simulink model "Part1_new"  (R2023b)
settings: Solver=ode23t  StartTime=0.0  StopTime=2  MaxStep=0.2  RelTol=1e-3
model workspace (MATLAB code in the model file):
  | m = 0.1;
  | d = 0.5;
  | k = 8;
libraries: fl_lib x29, nesl_utility x18
settings Model: Creator=oscar  LastModifiedBy=elliot
settings RTWCC: GPUComputeCapability=5.0

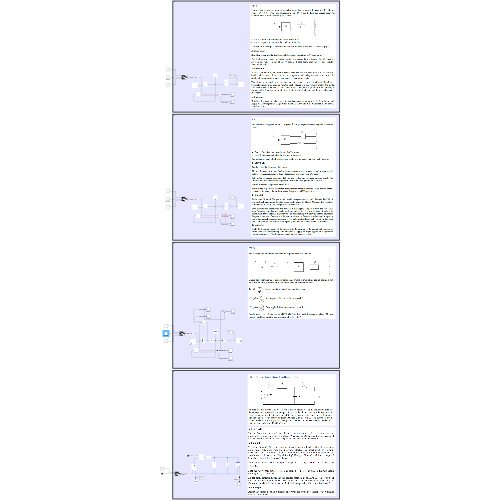
[thumbnail: Simulink's stored preview of the top-level diagram]
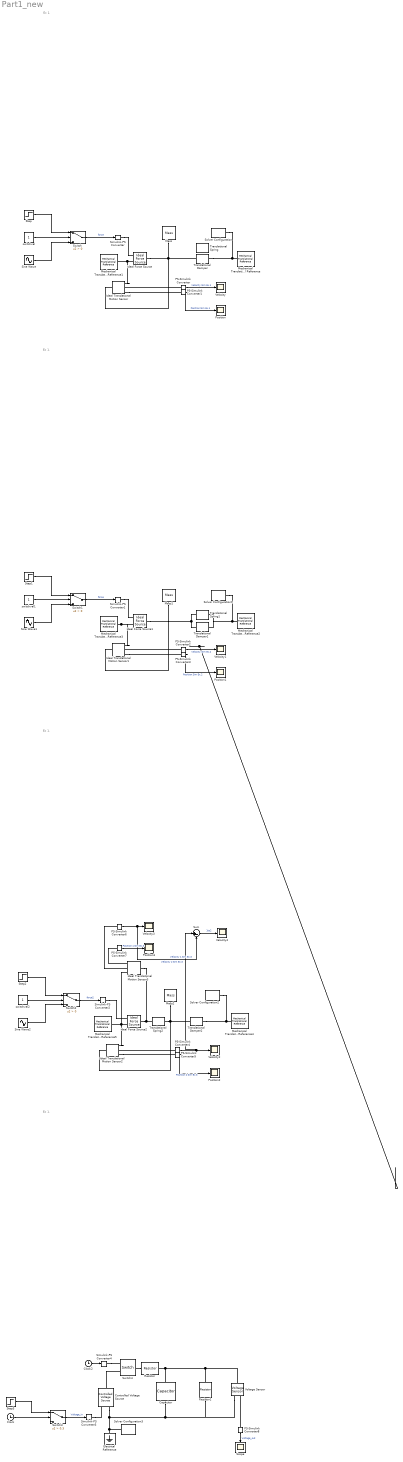
== system Part1_new ==
  note: Ex 1.
  note: Ex 1.
  note: Ex 1.
  note: Ex 1.
  Capacitor : fl_lib/Electrical/Electrical Elements/Capacitor  c=10 F  r=1e-6 Ohm  g=0 1/Ohm  i_specify=off  i_priority=None  i=0 A  i_nominal_specify=off  i_nominal_unit=A  i_nominal_value=1  v_specify=off  v_priority=None  v=0 V  v_nominal_specify=off  v_nominal_unit=V  v_nominal_value=1  vc_specify=off  vc_priority=High  vc=0 V  vc_nominal_specify=off  vc_nominal_unit=V  vc_nominal_value=1
  Clock : Clock
  Clock2 : Clock
  Controlled Voltage Source : fl_lib/Electrical/Electrical Sources/Controlled Voltage Source
  Electrical Reference : fl_lib/Electrical/Electrical Elements/Electrical Reference
  Ideal Force Source : fl_lib/Mechanical/Mechanical Sources/Ideal Force Source
  Ideal Force Source1 : fl_lib/Mechanical/Mechanical Sources/Ideal Force Source
  Ideal Force Source2 : fl_lib/Mechanical/Mechanical Sources/Ideal Force Source
  Ideal Translational Motion Sensor{,1..3} (4 alike) : fl_lib/Mechanical/Mechanical Sensors/Ideal Translational Motion Sensor  reference=foundation.enum.MeasurementReference.difference  acceleration_port=false  velocity_port=true  position_port=true  offset=0 m
  Mass : fl_lib/Mechanical/Translational Elements/Mass  mass=m kg  num_ports=foundation.enum.numPorts2.one  v_specify=off  v_priority=High  v=0 m/s  v_nominal_specify=off  v_nominal_unit=m/s  v_nominal_value=1  f_specify=off  f_priority=None  f=0 N  f_nominal_specify=off  f_nominal_unit=N  f_nominal_value=1
  Mass1 : fl_lib/Mechanical/Translational Elements/Mass  mass=m kg  num_ports=foundation.enum.numPorts2.one  v_specify=off  v_priority=High  v=0 m/s  v_nominal_specify=off  v_nominal_unit=m/s  v_nominal_value=1  f_specify=off  f_priority=None  f=0 N  f_nominal_specify=off  f_nominal_unit=N  f_nominal_value=1
  Mass2 : fl_lib/Mechanical/Translational Elements/Mass  mass=m kg  num_ports=foundation.enum.numPorts2.one  v_specify=off  v_priority=High  v=0 m/s  v_nominal_specify=off  v_nominal_unit=m/s  v_nominal_value=1  f_specify=off  f_priority=None  f=0 N  f_nominal_specify=off  f_nominal_unit=N  f_nominal_value=1
  Mechanical Translational Reference{,1..5} (6 alike) : fl_lib/Mechanical/Translational Elements/Mechanical Translational Reference
  PS-Simulink Converter{,1..8} (9 alike) : nesl_utility/PS-Simulink Converter  PhysicalDomain=network_engine_domain  SubClassName=ps_output  LeftPortType=input  RightPortType=output  PseudoPeriodic=off  Frequencies=[]  VectorFormat=inherit  Unit=inherit  AffineConversion=off
  Position{,1..3} (4 alike) : Scope
  Resistor : fl_lib/Electrical/Electrical Elements/Resistor  R=200 Ohm  i_specify=off  i_priority=None  i=0 A  i_nominal_specify=off  i_nominal_unit=A  i_nominal_value=1  v_specify=off  v_priority=None  v=0 V  v_nominal_specify=off  v_nominal_unit=V  v_nominal_value=1
  Resistor1 : fl_lib/Electrical/Electrical Elements/Resistor  R=200 Ohm  i_specify=off  i_priority=None  i=0 A  i_nominal_specify=off  i_nominal_unit=A  i_nominal_value=1  v_specify=off  v_priority=None  v=0 V  v_nominal_specify=off  v_nominal_unit=V  v_nominal_value=1
  Scope : Scope
  Simulink-PS Converter{,1,3..4} (4 alike) : nesl_utility/Simulink-PS Converter  PhysicalDomain=network_engine_domain  SubClassName=ps_input  LeftPortType=input  RightPortType=output  PseudoPeriodic=off  Frequencies=[]  NoiseDistribution=none  NoiseParameters=[]  Unit=1  AffineConversion=off  FilteringAndDerivatives=provide  SimscapeFilterOrder=1  InputFilterTimeConstant=0.001  UdotUserProvided=0
  Simulink-PS Converter2 : nesl_utility/Simulink-PS Converter  PhysicalDomain=network_engine_domain  SubClassName=ps_input  LeftPortType=input  RightPortType=output  PseudoPeriodic=off  Frequencies=[]  NoiseDistribution=none  NoiseParameters=[]  Unit=1  AffineConversion=off  FilteringAndDerivatives=filter  SimscapeFilterOrder=1  InputFilterTimeConstant=0.001  UdotUserProvided=0
  Sine Wave : Sin  Frequency=10  SampleTime=0
  Sine Wave1 : Sin  Frequency=10  SampleTime=0
  Sine Wave2 : Sin  Frequency=10  SampleTime=0
  Solver Configuration{,1..3} (4 alike) : nesl_utility/Solver Configuration  PhysicalDomain=network_engine_domain  SubClassName=solver  LeftPortType=input  RightPortType=generic  Tones=[]  Harmonics=[]  SimulateNoise=off  Profile=off  UseLocalSampling=off  EnableSwitchedLinearOptims=on  FrequencyDomain=off  UseCCode=off  RelTol=0.001  AbsTol=0.001  MinStep=1e-09  ToWorkspace=off  RevertToSquareIcSolve=off  NumHomotopyIterations=100  PhasorMode=off  PhasorModeNumHarmonics=1  ConsistencySolver=NEWTON_XTOL_AFTER_FTOL  IndexReductionMethod=DerivativeReplacement  DoDC=off  ResidualTolerance=1e-09  ConsistencyTolSource=GLOBAL  ConsistencyAbsTol=0.001  ConsistencyRelTol=0.001  ConsistencyTolFactor=0.001  UseLocalSolver=off  LocalSolverChoice=NE_BACKWARD_EULER_ADVANCER  ResolveIndetEquations=on  FunctionEvalNumThread=1  LocalSolverSampleTime=0.001  DoFixedCost=off  MaxNonlinIter=3  MaxModeIter=2  ComputeImpulses=off  ImpulseIterations=2  LinearAlgebra=auto  LinearAlgebraNumThread=0  EquationFormulation=NE_TIME_EF  DelaysMemoryBudget=1024  AutomaticFiltering=on  FilteringTimeConstant=0.001  PartitionStorageMethod=AS_NEEDED  PartitionMemoryBudget=1024  PartitionMethod=ROBUST  MultibodyUseLocalSolver=off  MultibodyLocalSolverChoice=ODE1  MultibodyLocalSolverSampleTime=0.001
  Step : Step  Time=0  SampleTime=0
  Step1 : Step  Time=0  SampleTime=0
  Step2 : Step  Time=0  SampleTime=0
  Step3 : Step  Time=0  After=12  SampleTime=0
  Sum : Sum  Inputs=|+-
  Switch : Switch  Criteria=u2 > Threshold  SaturateOnIntegerOverflow=off  InputSameDT=off
  Switch1 : Switch  Criteria=u2 > Threshold  SaturateOnIntegerOverflow=off  InputSameDT=off
  Switch2 : Switch  Criteria=u2 > Threshold  SaturateOnIntegerOverflow=off  InputSameDT=off
  Switch3 : Switch  Criteria=u2 > Threshold  Threshold=0.3  SaturateOnIntegerOverflow=off  InputSameDT=off
  Switch4 : fl_lib/Electrical/Electrical Elements/Switch  R_closed=0.0000001 Ohm  G_open=1e-8 1/Ohm  Threshold=0  i_specify=off  i_priority=None  i=0 A  i_nominal_specify=off  i_nominal_unit=A  i_nominal_value=1  v_specify=off  v_priority=None  v=0 V  v_nominal_specify=off  v_nominal_unit=V  v_nominal_value=1
  Translational Damper : fl_lib/Mechanical/Translational Elements/Translational Damper  D=d N*s/m  v_specify=off  v_priority=None  v=0 m/s  v_nominal_specify=off  v_nominal_unit=m/s  v_nominal_value=1  f_specify=off  f_priority=None  f=0 N  f_nominal_specify=off  f_nominal_unit=N  f_nominal_value=1
  Translational Damper1 : fl_lib/Mechanical/Translational Elements/Translational Damper  D=d N*s/m  v_specify=off  v_priority=None  v=0 m/s  v_nominal_specify=off  v_nominal_unit=m/s  v_nominal_value=1  f_specify=off  f_priority=None  f=0 N  f_nominal_specify=off  f_nominal_unit=N  f_nominal_value=1
  Translational Damper2 : fl_lib/Mechanical/Translational Elements/Translational Damper  D=d N*s/m  v_specify=off  v_priority=None  v=0 m/s  v_nominal_specify=off  v_nominal_unit=m/s  v_nominal_value=1  f_specify=off  f_priority=None  f=0 N  f_nominal_specify=off  f_nominal_unit=N  f_nominal_value=1
  Translational Spring : fl_lib/Mechanical/Translational Elements/Translational Spring  spr_rate=k N/m  v_specify=off  v_priority=None  v=0 m/s  v_nominal_specify=off  v_nominal_unit=m/s  v_nominal_value=1  f_specify=off  f_priority=None  f=0 N  f_nominal_specify=off  f_nominal_unit=N  f_nominal_value=1  x_specify=off  x_priority=High  x=0 m  x_nominal_specify=off  x_nominal_unit=m  x_nominal_value=1
  Translational Spring1 : fl_lib/Mechanical/Translational Elements/Translational Spring  spr_rate=k N/m  v_specify=off  v_priority=None  v=0 m/s  v_nominal_specify=off  v_nominal_unit=m/s  v_nominal_value=1  f_specify=off  f_priority=None  f=0 N  f_nominal_specify=off  f_nominal_unit=N  f_nominal_value=1  x_specify=off  x_priority=High  x=0 m  x_nominal_specify=off  x_nominal_unit=m  x_nominal_value=1
  Translational Spring2 : fl_lib/Mechanical/Translational Elements/Translational Spring  spr_rate=k N/m  v_specify=off  v_priority=None  v=0 m/s  v_nominal_specify=off  v_nominal_unit=m/s  v_nominal_value=1  f_specify=off  f_priority=None  f=0 N  f_nominal_specify=off  f_nominal_unit=N  f_nominal_value=1  x_specify=off  x_priority=High  x=0 m  x_nominal_specify=off  x_nominal_unit=m  x_nominal_value=1
  Velocity{,1..4} (5 alike) : Scope
  Voltage Sensor : fl_lib/Electrical/Electrical Sensors/Voltage Sensor
  switchval : Constant
  switchval1 : Constant
  switchval2 : Constant
  wires:
  PS-Simulink Converter/1 -> Velocity/1  "Velocity Sim Ex.1"
  PS-Simulink Converter1/1 -> Position/1  "Position Sim Ex.1"
  PS-Simulink Converter3/1 -> Position1/1  "Position Sim Ex.2"
  PS-Simulink Converter2/1 -> Velocity1/1  "Velocity Sim Ex.2"
  Switch/1 -> Simulink-PS Converter/1  "force"
  Sine Wave/1 -> Switch/3
  Step/1 -> Switch/1
  switchval/1 -> Switch/2
  switchval1/1 -> Switch1/2
  Step1/1 -> Switch1/1
  Switch1/1 -> Simulink-PS Converter1/1  "force"
  Sine Wave1/1 -> Switch1/3
  PS-Simulink Converter5/1 -> Position2/1  "Position 2 Sim Ex.3"
  PS-Simulink Converter4/1 -> Sum/1, Velocity2/1  "Velocity 2 Sim Ex.3"
  Switch2/1 -> Simulink-PS Converter2/1  "force2"
  Sine Wave2/1 -> Switch2/3
  switchval2/1 -> Switch2/2
  Step2/1 -> Switch2/1
  PS-Simulink Converter6/1 -> Sum/2, Velocity3/1  "Velocity 1 Sim Ex.3"
  PS-Simulink Converter7/1 -> Position3/1  "Position 1 Sim Ex.3"
  Clock/1 -> Switch3/2
  Step3/1 -> Switch3/1
  Switch3/1 -> Simulink-PS Converter3/1  "Voltage_in"
  PS-Simulink Converter8/1 -> Scope/1  "Voltage_out"
  Clock2/1 -> Simulink-PS Converter4/1
  Sum/1 -> Velocity4/1  "1to2"
  connections:
  Translational Damper/RConn1 -- Solver Configuration/RConn1 -- Mechanical Translational Reference/LConn1
  Mass/LConn1 -- Ideal Force Source/LConn1 -- Ideal Translational Motion Sensor/LConn1 -- Translational Damper/LConn1
  Ideal Force Source/RConn2 -- Ideal Translational Motion Sensor/RConn1 -- Mechanical Translational Reference1/LConn1
  Simulink-PS Converter/RConn1 -- Ideal Force Source/RConn1
  PS-Simulink Converter/LConn1 -- Ideal Translational Motion Sensor/RConn2
  Ideal Translational Motion Sensor/RConn3 -- PS-Simulink Converter1/LConn1
  Ideal Translational Motion Sensor1/LConn1 -- Mass1/LConn1 -- Ideal Force Source1/LConn1 -- Translational Damper1/LConn1 -- Translational Spring1/LConn1
  Mechanical Translational Reference3/LConn1 -- Ideal Translational Motion Sensor1/RConn1 -- Ideal Force Source1/RConn2
  Mechanical Translational Reference2/LConn1 -- Translational Damper1/RConn1 -- Translational Spring1/RConn1 -- Solver Configuration1/RConn1
  PS-Simulink Converter2/LConn1 -- Ideal Translational Motion Sensor1/RConn2
  Simulink-PS Converter1/RConn1 -- Ideal Force Source1/RConn1
  Ideal Translational Motion Sensor1/RConn3 -- PS-Simulink Converter3/LConn1
  Solver Configuration2/RConn1 -- Translational Damper2/RConn1 -- Mechanical Translational Reference4/LConn1
  Mass2/LConn1 -- Translational Damper2/LConn1 -- Ideal Translational Motion Sensor2/LConn1 -- Translational Spring2/RConn1
  Ideal Force Source2/RConn2 -- Ideal Translational Motion Sensor3/RConn1 -- Ideal Translational Motion Sensor2/RConn1 -- Mechanical Translational Reference5/LConn1
  PS-Simulink Converter4/LConn1 -- Ideal Translational Motion Sensor2/RConn2
  Ideal Translational Motion Sensor2/RConn3 -- PS-Simulink Converter5/LConn1
  Simulink-PS Converter2/RConn1 -- Ideal Force Source2/RConn1
  Ideal Force Source2/LConn1 -- Ideal Translational Motion Sensor3/LConn1 -- Translational Spring2/LConn1
  PS-Simulink Converter6/LConn1 -- Ideal Translational Motion Sensor3/RConn2
  Ideal Translational Motion Sensor3/RConn3 -- PS-Simulink Converter7/LConn1
  Simulink-PS Converter3/RConn1 -- Controlled Voltage Source/RConn1
  Controlled Voltage Source/RConn2 -- Resistor1/RConn1 -- Voltage Sensor/RConn2 -- Capacitor/RConn1 -- Solver Configuration3/RConn1 -- Electrical Reference/LConn1
  Resistor1/LConn1 -- Capacitor/LConn1 -- Resistor/RConn1 -- Voltage Sensor/LConn1
  Switch4/LConn1 -- Resistor/LConn1
  Controlled Voltage Source/LConn1 -- Switch4/RConn2
  PS-Simulink Converter8/LConn1 -- Voltage Sensor/RConn1
  Simulink-PS Converter4/RConn1 -- Switch4/RConn1
  ?
